simulink model "majatnick"  (R2016a)
settings: Solver=VariableStepAuto  StartTime=0.0  StopTime=150  RelTol=1e-3
values from neighbouring files (symbols this model uses):
  b = 0.1    [mm.m]
  g = 9.8    [mm.m]
  J = m*l^2    (= 1)    [mm.m]
  l = 1    [mm.m]
  m = 1    [mm.m]
libraries: simulink_extras x1
settings Model: Creator=Natasha  LastModifiedBy=Natasha

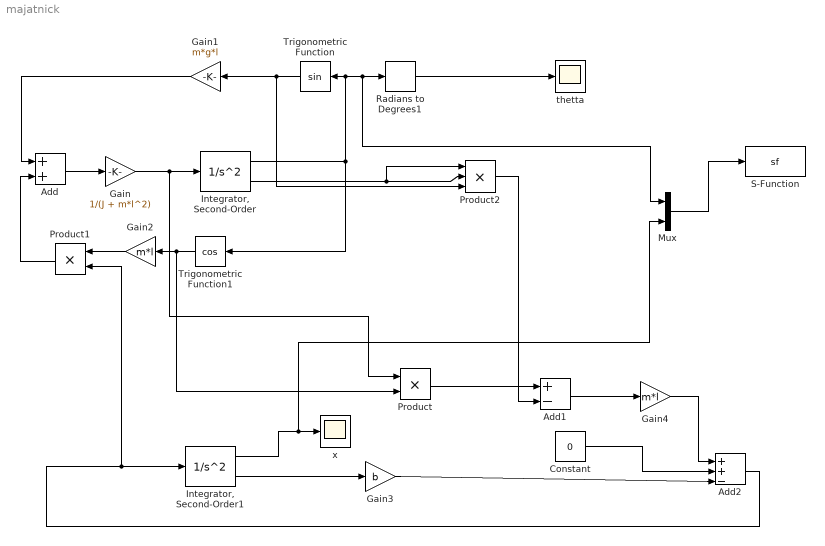
== system majatnick ==
  Add : Sum
  Add1 : Sum  Inputs=+-
  Add2 : Sum  Inputs=+|+-
  Constant : Constant  Value=0
  Gain : Gain  Gain=1/(J + m*l^2)
  Gain1 : Gain  Gain=m*g*l
  Gain2 : Gain  Gain=m*l
  Gain3 : Gain  Gain=b
  Gain4 : Gain  Gain=m*l
  "Integrator, Second-Order" : SecondOrderIntegrator  ICX=0.01  ICDXDT=0
  "Integrator, Second-Order1" : SecondOrderIntegrator  ICX=0.01
  Mux : Mux  Inputs=3
  Product : Product
  Product1 : Product
  Product2 : Product  Inputs=3
  Radians to Degrees1 : simulink_extras/Transformations/Radians to Degrees
  S-Function : S-Function  FunctionName=sf  Parameters=4 5  SFunctionDeploymentMode=off  EnableBusSupport=off
  Trigonometric Function : Trigonometry
  Trigonometric Function1 : Trigonometry  Operator=cos
  "thetta " : Scope
  "x " : Scope
  wires:
  Gain/1 -> Product/1, "Integrator, Second-Order"/1
  Gain1/1 -> Add/1
  Trigonometric Function/1 -> Product2/3, Gain1/1
  Add/1 -> Gain/1
  Gain2/1 -> Product1/1
  Trigonometric Function1/1 -> Product/2, Gain2/1
  Product1/1 -> Add/2
  Product/1 -> Add1/1
  "Integrator, Second-Order"/2 -> Product2/1, Product2/2
  Product2/1 -> Add1/2
  Add1/1 -> Gain4/1
  "Integrator, Second-Order1"/2 -> Gain3/1
  Gain4/1 -> Add2/1
  Gain3/1 -> Add2/3
  Constant/1 -> Add2/2
  Add2/1 -> "Integrator, Second-Order1"/1, Product1/2
  "Integrator, Second-Order"/1 -> Mux/1, Radians to Degrees1/1, Trigonometric Function/1, Trigonometric Function1/1
  "Integrator, Second-Order1"/1 -> Mux/3, "x "/1
  Mux/1 -> S-Function/1
  Radians to Degrees1/1 -> "thetta "/1
